simulink model "closed_loop_noise"  (Simulink 10.0)
settings: Solver=ode45  StartTime=0.0  StopTime=20  MaxStep=0.01  RelTol=1e-3  EnableMultiTasking=on
settings Model: Creator=akari  LastModifiedBy=linesLK
settings DataIOCC: LimitDataPoints=on  SignalLoggingSaveFormat=ModelDataLogs
settings OptimizationCC: ExpressionDepthLimit=2147483647
settings DebuggingCC: SolverPrmCheckMsg=warning  FcnCallInpInsideContextMsg=warning  StateNameClashWarn=warning
settings GRTTargetCC: GeneratePreprocessorConditionals=Disable all
settings ConfigComp: CovExternalEMLEnable=off

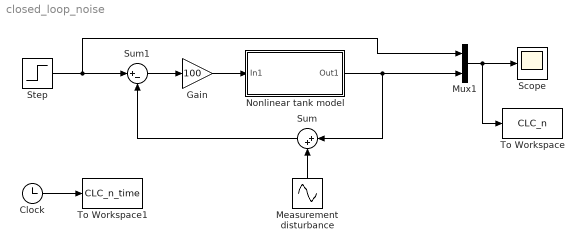
== system closed_loop_noise ==
  Clock : Clock
  Gain : Gain  Gain=100
  Measurement disturbance : Sin  Amplitude=0.1  Frequency=15  SampleTime=0
  Mux1 : Mux  Inputs=2
  Nonlinear tank model : Subsystem
  Scope : Scope
  Step : Step  Time=10  Before=0.6  After=1.8  SampleTime=0
  Sum : Sum  Inputs=|++
  Sum1 : Sum  Inputs=|+-
  To Workspace : ToWorkspace  VariableName=CLC_n  SampleTime=-1
  To Workspace1 : ToWorkspace  VariableName=CLC_n_time  SampleTime=-1
  wires:
  Sum1/1 -> Gain/1
  Gain/1 -> Nonlinear tank model/1(In1)
  Step/1 -> Sum1/1, Mux1/1
  Mux1/1 -> Scope/1, To Workspace/1
  Measurement disturbance/1 -> Sum/2
  Nonlinear tank model/1(Out1) -> Sum/1, Mux1/2
  Sum/1 -> Sum1/2
  Clock/1 -> To Workspace1/1

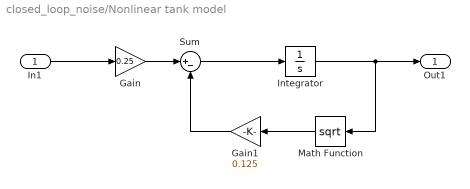
== system closed_loop_noise/Nonlinear tank model ==
  In1 : Inport
  Gain : Gain  Gain=0.25
  Gain1 : Gain  Gain=0.125
  Integrator : Integrator  InitialCondition=1
  Math Function : Math  Operator=sqrt  SaturateOnIntegerOverflow=on
  Sum : Sum  Inputs=|+-
  Out1 : Outport
  wires:
  Sum/1 -> Integrator/1
  Integrator/1 -> Math Function/1, Out1/1
  Math Function/1 -> Gain1/1
  Gain/1 -> Sum/1
  Gain1/1 -> Sum/2
  In1/1 -> Gain/1
